simulink model "Progetto_condizionatore_risposta"  (R2022a)
settings: Solver=VariableStepAuto  StartTime=0.0  StopTime=5*t_a  RelTol=1e-3
values from neighbouring files (symbols this model uses):
  A = [(-gamma_cs/C_c) (gamma_cs/C_c); (gamma_cs/C_s) -((gamma_cs/C_s)+(gamma_sa/C_s))]    [Progetto_condizionatore.m]
  B = [1/C_c; 0]    [Progetto_condizionatore.m]
  C = [0 1]    [Progetto_condizionatore.m]
  D = 0    [Progetto_condizionatore.m]
  temp_amb = 30    [Progetto_condizionatore.m]
  temp_des = 20    [Progetto_condizionatore.m]
  x0 = [23; 25]    [Progetto_condizionatore.m]
settings Model: Creator=Mattia  LastModifiedBy=decom

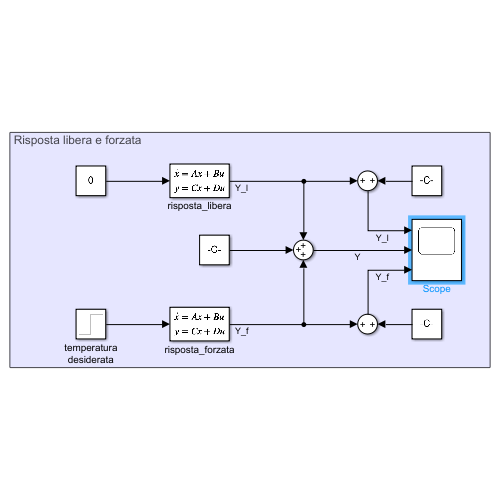
[thumbnail: Simulink's stored preview of the top-level diagram]
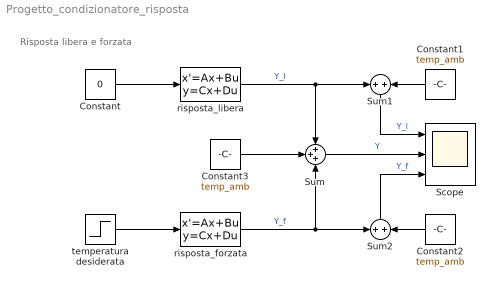
== system Progetto_condizionatore_risposta ==
  note: Risposta libera e forzata
  Constant : Constant  Value=0
  Constant1 : Constant  Value=temp_amb
  Constant2 : Constant  Value=temp_amb
  Constant3 : Constant  Value=temp_amb
  Scope : Scope  NumInputPorts=3
  Sum : Sum  Inputs=+++
  Sum1 : Sum
  Sum2 : Sum
  risposta_forzata : StateSpace  A=A  B=B  C=C  D=D  InitialCondition=0
  risposta_libera : StateSpace  A=A  B=B  C=C  D=D  InitialCondition=x0
  temperatura desiderata : Step  Time=0  After=temp_des  SampleTime=0
  wires:
  Constant/1 -> risposta_libera/1
  Sum/1 -> Scope/2  "Y"
  risposta_forzata/1 -> Sum/3, Sum2/1  "Y_f"
  risposta_libera/1 -> Sum1/1, Sum/1  "Y_l"
  temperatura desiderata/1 -> risposta_forzata/1
  Constant1/1 -> Sum1/2
  Sum1/1 -> Scope/1  "Y_l"
  Sum2/1 -> Scope/3  "Y_f"
  Constant2/1 -> Sum2/2
  Constant3/1 -> Sum/2
